simulink model "task2_2_1"  (R2020a)
settings: Solver=FixedStepAuto  StartTime=0.0  StopTime=60  FixedStep=0.01  RelTol=1e-3
settings Model: EnablePacing=on  PacingRate=10  Creator=dell  LastModifiedBy=dell

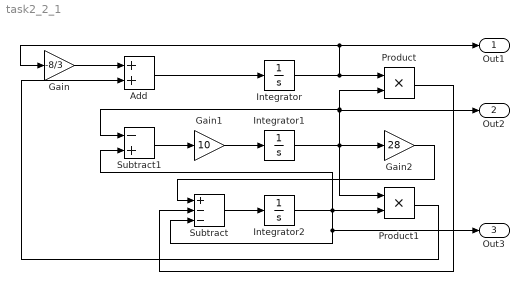
== system task2_2_1 ==
  Add : Sum
  Gain : Gain  Gain=-8/3
  Gain1 : Gain  Gain=10
  Gain2 : Gain  Gain=28
  Integrator : Integrator
  Integrator1 : Integrator
  Integrator2 : Integrator  InitialCondition=0.001
  Product : Product
  Product1 : Product
  Subtract : Sum  Inputs=+--
  Subtract1 : Sum  Inputs=-+
  Out1 : Outport
  Out2 : Outport  Port=2
  Out3 : Outport  Port=3
  wires:
  Integrator/1 -> Gain/1, Out1/1, Product/1
  Integrator1/1 -> Gain2/1, Subtract1/1, Product/2, Out2/1, Product1/1
  Integrator2/1 -> Subtract/3, Out3/1, Product1/2, Subtract1/2
  Gain/1 -> Add/1
  Product1/1 -> Add/2
  Add/1 -> Integrator/1
  Gain1/1 -> Integrator1/1
  Subtract1/1 -> Gain1/1
  Subtract/1 -> Integrator2/1
  Product/1 -> Subtract/2
  Gain2/1 -> Subtract/1
